simulink model "pr671_AM_DSB_TC_PLL"  (R2018b)
settings: Solver=VariableStepDiscrete  StartTime=0.0  StopTime=10  RelTol=1e-3  EnableMultiTasking=on
PreLoadFcn:
  | % pr671setup.m
  | % Инициализация параметров модели
  | fs = 48e3*10; %
  | fc = fs/5;
  | % параметры контура ФАПЧ
  | A = 1;       % амплитуда входного сигнала
  | T = 1/fs;    % период дискретизации
  | Kp = A/2;   % коэффициент усиления ФД
  | Bn = 1000; % шумовая полоса, Гц
  | Ko = 1;      % коэффициент усиления ГУН (нормирован к fs)
  | d = 0.707;  % демпинг фактор
  | % оценка коэффициентов ПФ
  | K1 = (4*d*Bn*T)/(Ko*Kp*(d+1/(4*d)));
  | K2 = (4*(Bn*T)^2)/(Ko*Kp*(d+1/4*d)^2);
StopFcn:
  | % Построение графика по завершении моделирования
  | figure(1);
  | plot(lo_freq.time,lo_freq.signals.values,'b');
  | hold on; grid on;
  | plot(tx_freq.time,tx_freq.signals.values,'r','linewidth',2);
  | xlabel('Время, с'); ylabel('Частота, Гц'); xlim([0 0.01]);
  | legend('Частота на выходе ГУН','Частота несущей');
libraries: dspmlti4 x6, dspvision x2, commsynccomp2 x2, dsparch4 x1
Description:
  | Software, Simulation Examples and Design Exercises Licence Agreement
  | 
  | This license agreement refers to the simulation examples, design exercises and files,
  | and associated software MATLAB and Simulink resources that accompany the book:
  | 
  |      Title: Software Defined Radio using MATLAB & Simulink and the RTL-SDR
  |      Published by Strathclyde Academic Media, 2015
  |      Authored by Robert W. Stewart, Kenneth W. Barlee, Dale S.W. Atkinson,
  |      and Louise H. Crockett
  | 
  | and made available as a download from, www.desktopSDR.com or variously acquired
  | by other means such as via USB storage, cloud storage, disk or any other electronic
  | or optical or magnetic storage mechanism. These files and associated software may
  | be used subject to the terms of agreement of the conditions below:
  | 
  |     Copyright © 2015 Robert W. Stewart, Kenneth W. Barlee, Dale S.W. Atkinson,
  |     and Louise H. Crockett
  |     All rights reserved.
  | 
  | Redistribution and use in source and binary forms, with or without modification, are
  | permitted provided that the following conditions are met:
  | 
  |    1.  Redistributions of source code must retain the above copyright notice, this list of
  |         conditions and the following disclaimer.
  | 
  |    2.  Redistributions in binary form must reproduce the above copyright notice, this
  |         list of conditions and the following disclaimer in the documentation and/or other
  |         materials provided with the distribution.
  | 
  |    3.  Neither the name of the copyright holder nor the names of its contributors may
  |         be used to endorse or promote products derived from this software without
  |         specific prior written permission.
  | 
  |    4.  In all cases, the software is, and all modifications and derivatives of the
  |         software shall be, licensed to you solely for use in conjunction with The
  |         MathWorks, Inc. products and service offerings.
  | 
  | THIS SOFTWARE IS PROVIDED BY THE COPYRIGHT HOLDERS AND CONTRIBUTORS
  | "AS IS" AND ANY EXPRESS OR IMPLIED WARRANTIES, INCLUDING, BUT NOT LIMITED
  | TO, THE IMPLIED WARRANTIES OF MERCHANTABILITY AND FITNESS FOR A
  | PARTICULAR PURPOSE ARE DISCLAIMED. IN NO EVENT SHALL THE COPYRIGHT
  | HOLDER OR CONTRIBUTORS BE LIABLE FOR ANY DIRECT, INDIRECT, INCIDENTAL,
  | SPECIAL, EXEMPLARY, OR CONSEQUENTIAL DAMAGES (INCLUDING, BUT NOT
  | LIMITED TO, PROCUREMENT OF SUBSTITUTE GOODS OR SERVICES; LOSS OF USE,
  | DATA, OR PROFITS; OR BUSINESS INTERRUPTION) HOWEVER CAUSED AND ON ANY
  | THEORY OF LIABILITY, WHETHER IN CONTRACT, STRICT LIABILITY, OR TORT
  | (INCLUDING NEGLIGENCE OR OTHERWISE) ARISING IN ANY WAY OUT OF THE USE
  | OF THIS SOFTWARE, EVEN IF ADVISED OF THE POSSIBILITY OF SUCH DAMAGE.
  | 
  | 
  | Audio Tracks used in Simulations Examples and Design Exercises
  | 
  | The music and vocal files used within the Examples files and software within the book
  | were variously written, arranged, performed, recorded and produced by Garrey Rice,
  | Adam Struth, Jamie Struth, Iain Thistlethwaite and also Marshall Craigmyle who
  | collectively, and individually where appropriate, assert and retain all of their copyright,
  | performance and artistic rights. Permission to use and reproduce this music is
  | granted for all purposes associated with MATLAB and Simulink software and the
  | simulation examples and design exercises files that accompany this book. Requests to
  | use the music for any other purpose should be directed to: info@desktopSDR.com.
  | For information on music track names, full credits, and links to the musicians please
  | refer to www.desktopSDR.com/more/audio.
settings Model: Creator=desktopSDR Team  LastModifiedBy=Григорий Фокин
settings DataIOCC: SaveFormat=Array  SaveOutput=off  SignalLogging=off  SaveTime=off
settings OptimizationCC: DefaultParameterBehavior=Inlined  LifeSpan=inf
settings DebuggingCC: ReadBeforeWriteMsg=DisableAll  WriteAfterWriteMsg=DisableAll  WriteAfterReadMsg=DisableAll  UnderspecifiedInitializationDetection=Classic  MergeDetectMultiDrivingBlocksExec=none  SolverPrmCheckMsg=warning  MultiTaskDSMMsg=none  ParameterPrecisionLossMsg=none  SFUnexpectedBacktrackingDiag=warning  SFNoUnconditionalDefaultTransitionDiag=warning  SFExecutionAtInitializationDiag=none
settings HardwareCC: ProdBitPerPointer=32  ProdBitPerSizeT=32  ProdBitPerPtrDiffT=32  ProdLargestAtomicFloat=None  ProdIntDivRoundTo=Undefined  ProdEndianess=Unspecified  ProdWordSize=32  ProdHWDeviceType=32-bit Generic
settings ModelReferenceCC: UpdateModelReferenceTargets=IfOutOfDate  PropagateSignalLabelsOutOfModel=off
settings SFSimCC: SFSimEcho=off  SimUseLocalCustomCode=off
settings RTWCC: RTWUseLocalCustomCode=off
settings CodeAppCC: StateflowObjectComments=on
settings GRTTargetCC: TargetLangStandard=C89/C90 (ANSI)  GeneratePreprocessorConditionals=Disable all
settings ConfigComp: CovMetricSettings=dw  CovHtmlReporting=on  CovSaveCumulativeToWorkspaceVar=on  CovSaveSingleToWorkspaceVar=on  CovExternalEMLEnable=off  CovSFcnEnable=off

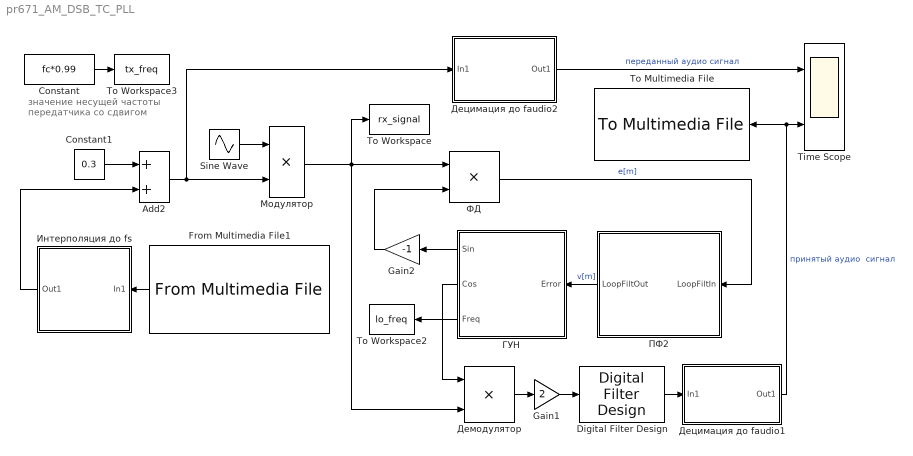
== system pr671_AM_DSB_TC_PLL ==
  note: значение
      | несущей частоты
      | передатчика со сдвигом
  Add2 : Sum
  Constant : Constant  Value=fc*0.99  SampleTime=1/fs
  Constant1 : Constant  Value=0.3  SampleTime=1/fs
  Digital Filter Design : dsparch4/Digital Filter Design  mwdsp_browser_bugfix_var=off
  From Multimedia File1 : dspvision/From Multimedia File  inputFilename=C:\Users\Григорий Фокин\Documents\MATLAB\sut_study\dcsdr\audio_sources\music1_mono48kHz.wav  loop=on  numPlays=inf  outputStreams=Audio only  videoDataType=single  audioDataType=double  inheritSampleTime=on  userDefinedSampleTime=1/30  noAudioOutput=off  isIntensityVideo=off  fourcc=RGB  colorVideoFormat=Separate color signals  outputEOF=off  dataOrg=Column-major  audioFrameSize=600  computeAudioFrameSize=off  outSamplingMode=Frame based
      settings: SourceProductBaseCode=VP
  Gain1 : Gain  Gain=2
  Gain2 : Gain  Gain=-1
  Sine Wave : Sin  Frequency=2*pi*fc*0.99  Phase=pi/5  SampleTime=1/fs
  Time Scope : Scope  NumInputPorts=2
  To Multimedia File : dspvision/To Multimedia File  outputFilename=demod_audio.wav  streamSelection=Audio only  videoCompressor=None (uncompressed)  audioCompressor=None (uncompressed)  imagePorts=Separate color signals  fileType=WAV  audioDatatype=16-bit integer  fourcc=RGB  videoQuality=75  mj2000CompFactor=10
      settings: SourceProductName=Computer Vision System Toolbox  SourceProductBaseCode=VP
  To Workspace : ToWorkspace  VariableName=rx_signal  SaveFormat=Structure With Time  SampleTime=-1
  To Workspace2 : ToWorkspace  VariableName=lo_freq  SaveFormat=Structure With Time  SampleTime=-1
  To Workspace3 : ToWorkspace  VariableName=tx_freq  SaveFormat=Structure With Time  SampleTime=-1
  ГУН : Subsystem  mask(Quadratude VCO){fq=fc, sensitivity=Ko*fs}
      mask prompts: fq "Quiescent Frequency (Hz)"; sensitivity "Sensitivity (Hz/V)"
      mask help: This VCO provides both cosine and sine outputs. The quiescent frequency and sensitivity of the VCO can be defined via the mask (and these apply to both sine and cosine outputs). The block also provides the instantaneous frequency as an output.
  Демодулятор : Product
  Децимация до faudio1 : Subsystem
  Децимация до faudio2 : Subsystem
  Интерполяция до fs : Subsystem
  Модулятор : Product
  ПФ2 : Subsystem  mask(Loop Filter (Type 2)){K1=K1, K2=K2}
      mask prompts: K1 "K1 (proportional path)"; K2 "K2 (integral path)"
      mask help: This loop filter contains two paths: a proportional path with scaling coefficient K1, and an integral path with scaling coefficient K2.
  ФД : Product
  wires:
  Sine Wave/1 -> Модулятор/1
  Модулятор/1 -> To Workspace/1, Демодулятор/2, ФД/1
  Демодулятор/1 -> Gain1/1
  ФД/1 -> ПФ2/1(LoopFiltIn)  "e[m]"
  Gain2/1 -> ФД/2
  ГУН/3(Freq) -> To Workspace2/1
  Constant/1 -> To Workspace3/1
  Constant1/1 -> Add2/1
  Децимация до faudio1/1(Out1) -> Time Scope/2, To Multimedia File/1  "принятый аудио  сигнал"
  Digital Filter Design/1 -> Децимация до faudio1/1(In1)
  ГУН/2(Cos) -> Демодулятор/1
  Add2/1 -> Децимация до faudio2/1(In1), Модулятор/2
  Децимация до faudio2/1(Out1) -> Time Scope/1  "переданный аудио сигнал"
  Gain1/1 -> Digital Filter Design/1
  ГУН/1(Sin) -> Gain2/1
  Интерполяция до fs/1(Out1) -> Add2/2
  From Multimedia File1/1 -> Интерполяция до fs/1(In1)
  ПФ2/1(LoopFiltOut) -> ГУН/1(Error)  "v[m]"

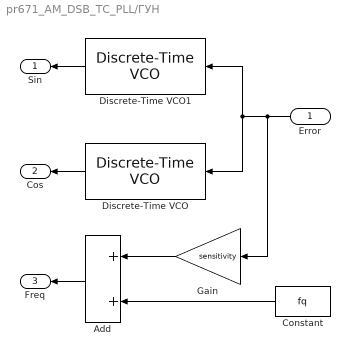
== system pr671_AM_DSB_TC_PLL/ГУН ==
  Error : Inport
  Add : Sum
  Constant : Constant  Value=fq  SampleTime=1/fs
  Discrete-Time VCO : commsynccomp2/Discrete-Time VCO  Ac=1  Fc=fq  Kc=sensitivity  Ph=pi/2  ts=1/fs
      settings: SourceProductName=Communications System Toolbox  SourceProductBaseCode=CM
  Discrete-Time VCO1 : commsynccomp2/Discrete-Time VCO  Ac=1  Fc=fq  Kc=sensitivity  Ph=0  ts=1/fs
      settings: SourceProductName=Communications System Toolbox  SourceProductBaseCode=CM
  Gain : Gain  Gain=sensitivity
  Sin : Outport
  Cos : Outport  Port=2
  Freq : Outport  Port=3
  wires:
  Discrete-Time VCO1/1 -> Sin/1
  Discrete-Time VCO/1 -> Cos/1
  Error/1 -> Discrete-Time VCO/1, Discrete-Time VCO1/1, Gain/1
  Gain/1 -> Add/1
  Constant/1 -> Add/2
  Add/1 -> Freq/1

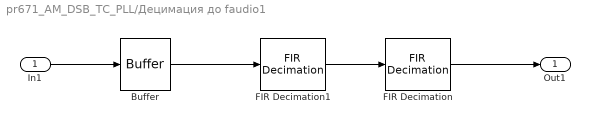
== system pr671_AM_DSB_TC_PLL/Децимация до faudio1 ==
  In1 : Inport
  Buffer : Buffer
  FIR Decimation : dspmlti4/FIR Decimation  FilterSource=Dialog parameters  h=fir1(35,1/5)  D=5  filtStruct=Direct form  FilterObject=Hm_firdecim  InputProcessing=Columns as channels (frame based)  framing=Allow multirate processing  inputOffset=0  outputBufInitCond=0  roundingMode=Floor  overflowMode=off  firstCoeffDataTypeStr=Inherit: Same word length as input  firstCoeffMin=[]  firstCoeffMax=[]  firstCoeffLastDataTypeStr=Inherit: Same word length as input  outputDataTypeStr=Inherit: Same as accumulator  outputMin=[]  outputMax=[]  outputLastDataTypeStr=Inherit: Same as accumulator
  FIR Decimation1 : dspmlti4/FIR Decimation  FilterSource=Dialog parameters  h=fir1(35,1/2)  D=2  filtStruct=Direct form  FilterObject=Hm_firdecim  InputProcessing=Columns as channels (frame based)  framing=Allow multirate processing  inputOffset=0  outputBufInitCond=0  roundingMode=Floor  overflowMode=off  firstCoeffDataTypeStr=Inherit: Same word length as input  firstCoeffMin=[]  firstCoeffMax=[]  firstCoeffLastDataTypeStr=Inherit: Same word length as input  outputDataTypeStr=Inherit: Same as accumulator  outputMin=[]  outputMax=[]  outputLastDataTypeStr=Inherit: Same as accumulator
  Out1 : Outport
  wires:
  FIR Decimation/1 -> Out1/1
  FIR Decimation1/1 -> FIR Decimation/1
  Buffer/1 -> FIR Decimation1/1
  In1/1 -> Buffer/1

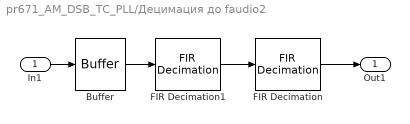
== system pr671_AM_DSB_TC_PLL/Децимация до faudio2 ==
  In1 : Inport
  Buffer : Buffer
  FIR Decimation : dspmlti4/FIR Decimation  FilterSource=Dialog parameters  h=fir1(35,1/5)  D=5  filtStruct=Direct form  FilterObject=Hm_firdecim  InputProcessing=Columns as channels (frame based)  framing=Allow multirate processing  inputOffset=0  outputBufInitCond=0  roundingMode=Floor  overflowMode=off  firstCoeffDataTypeStr=Inherit: Same word length as input  firstCoeffMin=[]  firstCoeffMax=[]  firstCoeffLastDataTypeStr=Inherit: Same word length as input  outputDataTypeStr=Inherit: Same as accumulator  outputMin=[]  outputMax=[]  outputLastDataTypeStr=Inherit: Same as accumulator
  FIR Decimation1 : dspmlti4/FIR Decimation  FilterSource=Dialog parameters  h=fir1(35,1/2)  D=2  filtStruct=Direct form  FilterObject=Hm_firdecim  InputProcessing=Columns as channels (frame based)  framing=Allow multirate processing  inputOffset=0  outputBufInitCond=0  roundingMode=Floor  overflowMode=off  firstCoeffDataTypeStr=Inherit: Same word length as input  firstCoeffMin=[]  firstCoeffMax=[]  firstCoeffLastDataTypeStr=Inherit: Same word length as input  outputDataTypeStr=Inherit: Same as accumulator  outputMin=[]  outputMax=[]  outputLastDataTypeStr=Inherit: Same as accumulator
  Out1 : Outport
  wires:
  In1/1 -> Buffer/1
  Buffer/1 -> FIR Decimation1/1
  FIR Decimation1/1 -> FIR Decimation/1
  FIR Decimation/1 -> Out1/1

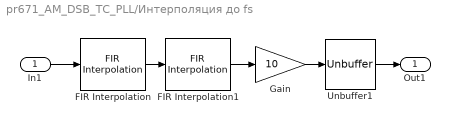
== system pr671_AM_DSB_TC_PLL/Интерполяция до fs ==
  In1 : Inport
  FIR Interpolation : dspmlti4/FIR Interpolation  FilterSource=Dialog parameters  h=fir1(35,1/5)  L=5  FilterObject=Hm_firinterp  InputProcessing=Columns as channels (frame based)  framing=Allow multirate processing  outputBufInitCond=0  roundingMode=Floor  overflowMode=off  firstCoeffDataTypeStr=Inherit: Same word length as input  firstCoeffMin=[]  firstCoeffMax=[]  firstCoeffLastDataTypeStr=Inherit: Same word length as input  outputDataTypeStr=Inherit: Same as accumulator  outputMin=[]  outputMax=[]  outputLastDataTypeStr=Inherit: Same as accumulator
      settings: SourceProductName=DSP System Toolbox
  FIR Interpolation1 : dspmlti4/FIR Interpolation  FilterSource=Dialog parameters  h=fir1(35,1/2)  L=2  FilterObject=Hm_firinterp  InputProcessing=Columns as channels (frame based)  framing=Allow multirate processing  outputBufInitCond=0  roundingMode=Floor  overflowMode=off  firstCoeffDataTypeStr=Inherit: Same word length as input  firstCoeffMin=[]  firstCoeffMax=[]  firstCoeffLastDataTypeStr=Inherit: Same word length as input  outputDataTypeStr=Inherit: Same as accumulator  outputMin=[]  outputMax=[]  outputLastDataTypeStr=Inherit: Same as accumulator
      settings: SourceProductName=DSP System Toolbox
  Gain : Gain  Gain=10
  Unbuffer1 : Unbuffer
  Out1 : Outport
  wires:
  Unbuffer1/1 -> Out1/1
  Gain/1 -> Unbuffer1/1
  In1/1 -> FIR Interpolation/1
  FIR Interpolation1/1 -> Gain/1
  FIR Interpolation/1 -> FIR Interpolation1/1

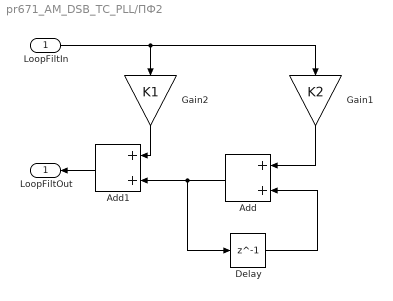
== system pr671_AM_DSB_TC_PLL/ПФ2 ==
  LoopFiltIn : Inport
  Add : Sum
  Add1 : Sum
  Delay : Delay  DelayLength=1
  Gain1 : Gain  Gain=K2
  Gain2 : Gain  Gain=K1
  LoopFiltOut : Outport
  wires:
  Add1/1 -> LoopFiltOut/1
  Delay/1 -> Add/2
  Add/1 -> Delay/1, Add1/2
  LoopFiltIn/1 -> Gain1/1, Gain2/1
  Gain2/1 -> Add1/1
  Gain1/1 -> Add/1
